simulink library "rfmathmodels1"  (Simulink 6.0)
settings: Solver=ode45  SolverMode=SingleTasking  StartTime=0.0  StopTime=10.0  RelTol=1e-3
undefined symbols (not defined in the file or in its folder): c1, inputGain, kT, method, outputGain
libraries: rfprivate1 x6, dspsigattribs x4, dspmathops x2, dsparch3 x1
settings Model: RequirementInfo=9  CovMetricSettings=d  Creator=tdelve  LastModifiedBy=rzeng  ExtModeAutoUpdateStatusClock=off  ProdHWDeviceType=Specified
settings DataIOCC: SignalLoggingName=logsOut
settings OptimizationCC: BooleanDataType=off
settings DebuggingCC: CheckExecutionContextPreStartOutputMsg=on  CheckExecutionContextRuntimeOutputMsg=on  SolverPrmCheckMsg=none
settings HardwareCC: ProdHWDeviceType=Specified
settings ModelReferenceCC: UpdateModelReferenceTargets=IfOutOfDate
settings SFSimCC: SFSimApplyToAllLibs=on  SFSimBuildMode=Incremental

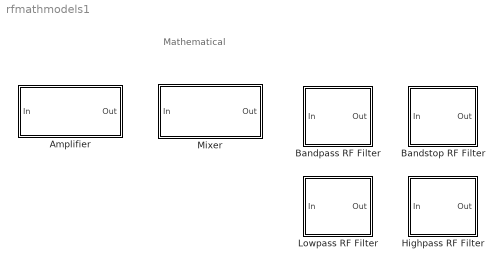
== system rfmathmodels1 ==
  note: Mathematical
  Amplifier : Subsystem  PropExecContextAcrossSSBoundary=on  mask(Amplifier){model_select=Linear, linGaindB=0, GindB=0, iip3=30, am2pm=0, amam=[2.1587 1.1517], ampm=[4.0033 9.1040], x=[8.1081 1.5413 6.5202 -0.0718], y=[4.6645 2.0965 10.88 -0.003], p=0.5, GoutdB=0, vsat=1, method_select=Noise factor, ntemp=290, nfigure=3.01, nfactor=2, seed=67987}
      mask prompts: model_select "Method:"; linGaindB "Linear gain (dB):"; GindB "Input scaling (dB):"; iip3 "IIP3 (dBm):"; am2pm "AM/PM conversion (degrees per dB):"; amam "AM/AM parameters [alpha beta]:"; ampm "AM/PM parameters [alpha beta]:"; x "AM/AM parameters [x1 x2 x3 x4]:"; y "AM/PM parameters [y1 y2 y3 y4]:"; p "Smoothness factor:"; GoutdB "Output scaling (dB):"; vsat "Output saturation level:"; method_select "Specification method:"; ntemp "Noise temperature (K):"; nfigure "Noise figure (dB):"; nfactor "Noise factor:"; seed "Initial seed:"
      mask help:
      | Complex baseband model of amplifier with noise.
      |
      | In addition to Linear amplifier, this block has five different methods to model the nonlinear amplifier.
      |
      | Two of the nonlinear methods (Cubic Polynomial and Hyperbolic Tangent) fit curves to measured data provided by the gain and third order intercept point (IIP3) parameters.
      |
      | The other three nonlinear methods use models originated by Saleh, Ghorbani, and Rapp.  The Saleh and Ghorbani models are based on normalized nonlinear transfer functions.  Use the Input scaling and Output scaling parameters to adjust signal levels up or down from their normalized values.
      |
      | The amount of noise added to the output signal may be specified either in terms of noise temperature, noise figure, or noise factor.
      mask init:
      | [c1, method, inputGain, outputGain, kT] = rfblksmathamp1(gcb, 'rfInit');
      mask Help: helpview(rfbhelp)
      mask StyleString: popup(Linear|Cubic polynomial|Hyperbolic tangent|Saleh model|Ghorbani model|Rapp model),edit,edit,edit,edit,edit,edit,edit,edit,edit,edit,edit,popup(Noise temperature|Noise figure|Noise factor),edit,edit,edit,edit
      mask CallbackString: rfblksmathamp1(gcb, 'rfModel');||||||||||||rfblksmathamp1(gcb, 'rfMethod');||||
      mask Display: disp('Amplifier');
  Bandpass RF Filter : Subsystem  PropExecContextAcrossSSBoundary=on  mask(Bandpass RF Filter){method=Butterworth, filttype=Bandpass, N=3, flo=1.9998e9, fhi=2.0002e9, Rp=1, Rs=10, MaxLength=32, Fc=2e9, Ts=1e-6}
      mask prompts: method "Design method:"; filttype "Filter type:"; N "Filter order:"; flo "Lower passband edge frequency (Hz):"; fhi "Upper passband edge frequency (Hz):"; Rp "Passband ripple in dB:"; Rs "Stopband attenuation in dB:"; MaxLength "Max length of impulse response:"; Fc "Center frequency (Hz):"; Ts "Sample time (s):"
      mask help: Design one of several standard bandpass filters, implemented in baseband equivalent complex form.
      mask init:
      | load rfblksfiltericons;
      | h = [yline+2 yline ywav];
      | w = [xline xline xwav];
      | model = rfblksfilters1(gcb, 'rfInit');
      mask Help: helpview(rfbhelp)
      mask StyleString: popup(Butterworth|Chebyshev I|Chebyshev II|Elliptic|Bessel),popup(Bandpass),edit,edit,edit,edit,edit,edit,edit,edit
      mask CallbackString: rfblksfilters1(gcb);|rfblksfilters1(gcb);||||||||
      mask Display: plot(w,h)
  Bandstop RF Filter : Subsystem  PropExecContextAcrossSSBoundary=on  mask(Bandstop RF Filter){method=Butterworth, filttype=Bandstop, N=3, flo=1.9998e9, fhi=2.0002e9, Rp=1, Rs=10, MaxLength=32, Fc=2e9, Ts=1e-6}
      mask prompts: method "Design method:"; filttype "Filter type:"; N "Filter order:"; flo "Lower passband edge frequency (Hz):"; fhi "Upper passband edge frequency (Hz):"; Rp "Passband ripple in dB:"; Rs "Stopband attenuation in dB:"; MaxLength "Max length of impulse response:"; Fc "Center frequency (Hz):"; Ts "Sample time (s):"
      mask help: Design one of several standard bandstop filters, implemented in baseband equivalent complex form.
      mask init:
      | load rfblksfiltericons;
      | h = [yline+1 ywav];
      | w = [xline xwav];
      | model = rfblksfilters1(gcb, 'rfInit');
      mask Help: helpview(rfbhelp)
      mask StyleString: popup(Butterworth|Chebyshev I|Chebyshev II|Elliptic|Bessel),popup(Bandstop),edit,edit,edit,edit,edit,edit,edit,edit
      mask CallbackString: rfblksfilters1(gcb);|rfblksfilters1(gcb);||||||||
      mask Display: plot(w,h)
  Highpass RF Filter : Subsystem  PropExecContextAcrossSSBoundary=on  mask(Highpass RF Filter){method=Butterworth, filttype=Highpass, N=3, flo=1.9998e9, fhi=2.0002e9, Rp=1, Rs=10, MaxLength=32, Fc=2e9, Ts=1e-6}
      mask prompts: method "Design method:"; filttype "Filter type:"; N "Filter order:"; flo "Passband edge frequency (Hz):"; fhi "(unused)"; Rp "Passband ripple in dB:"; Rs "Stopband attenuation in dB:"; MaxLength "Max length of impulse response:"; Fc "Center frequency:"; Ts "Sample time (s):"
      mask help: Design one of several standard highpass filters, implemented in baseband equivalent complex form.
      mask init:
      | load rfblksfiltericons;
      | h = [yline yline+1 ywav];
      | w = [xline xline xwav];
      | model = rfblksfilters1(gcb, 'rfInit');
      mask Help: helpview(rfbhelp)
      mask StyleString: popup(Butterworth|Chebyshev I|Chebyshev II|Elliptic|Bessel),popup(Highpass),edit,edit,edit,edit,edit,edit,edit,edit
      mask CallbackString: rfblksfilters1(gcb);|rfblksfilters1(gcb);||||||||
      mask Display: plot(w,h)
  Lowpass RF Filter : Subsystem  PropExecContextAcrossSSBoundary=on  mask(Lowpass RF Filter){method=Butterworth, filttype=Lowpass, N=3, flo=1.9998e9, fhi=2.0002e9, Rp=1, Rs=10, MaxLength=32, Fc=2e9, Ts=1e-6}
      mask prompts: method "Design method:"; filttype "Filter type:"; N "Filter order:"; flo "Passband edge frequency (Hz):"; fhi "(unused)"; Rp "Passband ripple in dB:"; Rs "Stopband attenuation in dB:"; MaxLength "Max length of impulse response:"; Fc "Center frequency (Hz):"; Ts "Sample time (s):"
      mask help: Design one of several standard lowpass filters, implemented in baseband equivalent complex form.
      mask init:
      | load rfblksfiltericons;
      | h = [yline+2 yline+1 ywav];
      | w = [xline xline xwav];
      | model = rfblksfilters1(gcb, 'rfInit');
      mask Help: helpview(rfbhelp)
      mask StyleString: popup(Butterworth|Chebyshev I|Chebyshev II|Elliptic|Bessel),popup(Lowpass),edit,edit,edit,edit,edit,edit,edit,edit
      mask CallbackString: rfblksfilters1(gcb);|rfblksfilters1(gcb);||||||||
      mask Display: plot(w,h)
  Mixer : Subsystem  PropExecContextAcrossSSBoundary=on  mask(Mixer){loss=0, PhNs=-120, Fo=100, seed=2137}
      mask prompts: loss "Conversion loss (dB):"; PhNs "Phase noise level (dBc/Hz):"; Fo "Frequency offset (Hz):"; seed "Initial seed:"
      mask help:
      | Complex baseband model of mixer with phase noise.
      |
      | The phase noise of this block characterized by a 1/f slope.  The level of the spectrum is specified by the noise power contained in a one hertz bandwidth offset from the carrier by a certain frequency.
      mask init:
      | c1 = 10^(-loss/20);
      | 
      | if PhNs>0,
      | 	error('Phase noise level should be negative.');
      | end
      | num = sqrt(2*pi*Fo*10^((PhNs)/10));
      | if num>.1,
      | 	warning('Current parameters in phase noise block may produce inaccurate results.');
      | end
      | num_taps = 64;
      | den = zeros(1,num_taps);
      | den(1) = 1;
      | for idx = 2:num_taps
      |    den(idx) = (idx - 2.5) * den(idx-1) / (idx-1);
      | end
      mask Help: helpview(rfbhelp)
      mask Display: disp('Mixer');

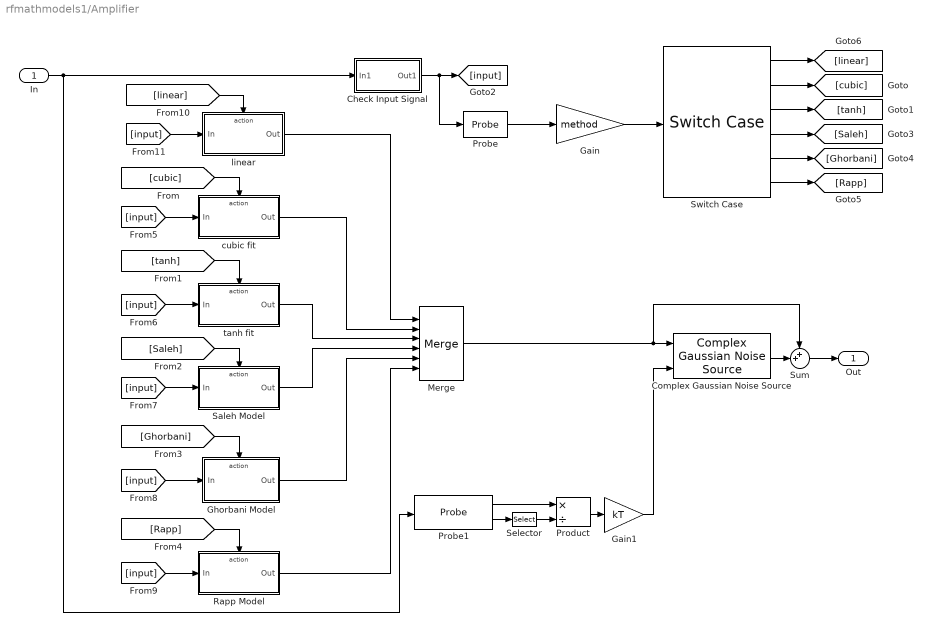
== system rfmathmodels1/Amplifier ==
  In : Inport  LatchInput=off
  Check Input Signal : Subsystem  PropExecContextAcrossSSBoundary=on
      mask Display: disp('Check\nInput Signal');
  Complex Gaussian Noise Source : rfprivate1/Complex Gaussian Noise Source
  Gain : Gain  Gain=method  SaturateOnIntegerOverflow=on
  Gain1 : Gain  Gain=kT  SaturateOnIntegerOverflow=on
  Ghorbani Model : Subsystem  TreatAsAtomicUnit=on  PropExecContextAcrossSSBoundary=on
  Merge : Merge  Inputs=6
  Probe : Probe  ProbeWidth=off  ProbeSampleTime=off
  Probe1 : Probe  ProbeComplexSignal=off
  Product : Product  Inputs=*/  SaturateOnIntegerOverflow=on  InputSameDT=on
  Rapp Model : Subsystem  TreatAsAtomicUnit=on  PropExecContextAcrossSSBoundary=on
  Saleh Model : Subsystem  TreatAsAtomicUnit=on  PropExecContextAcrossSSBoundary=on
  Selector : Selector  InputPortWidth=2
  Sum : Sum  Inputs=++|
  Switch Case : SwitchCase  CaseConditions={0 1 2 3 4 5}  CaseShowDefault=off
  cubic fit : Subsystem  TreatAsAtomicUnit=on  PropExecContextAcrossSSBoundary=on
  linear : Subsystem  TreatAsAtomicUnit=on  PropExecContextAcrossSSBoundary=on
  tanh fit : Subsystem  TreatAsAtomicUnit=on  PropExecContextAcrossSSBoundary=on
  Out : Outport
  wires:
  Merge/1 -> Complex Gaussian Noise Source/1, Sum/1
  Selector/1 -> Product/2
  Probe1/2 -> Selector/1
  Gain1/1 -> Complex Gaussian Noise Source/2
  Product/1 -> Gain1/1
  Probe1/1 -> Product/1
  Sum/1 -> Out/1
  Gain/1 -> Switch Case/1
  [cubic] -> cubic fit/Action
  [tanh] -> tanh fit/Action
  In/1 -> Probe1/1, Check Input Signal/1(In1)
  Check Input Signal/1(Out1) -> [input], Probe/1
  [Rapp] -> Rapp Model/Action
  [Ghorbani] -> Ghorbani Model/Action
  [Saleh] -> Saleh Model/Action
  [input] -> cubic fit/1(In)
  [input] -> Rapp Model/1(In)
  [input] -> Ghorbani Model/1(In)
  [input] -> Saleh Model/1(In)
  [input] -> tanh fit/1(In)
  Probe/1 -> Gain/1
  Rapp Model/1(Out) -> Merge/6
  [linear] -> linear/Action
  [input] -> linear/1(In)
  Ghorbani Model/1(Out) -> Merge/5
  Saleh Model/1(Out) -> Merge/4
  tanh fit/1(Out) -> Merge/3
  cubic fit/1(Out) -> Merge/2
  linear/1(Out) -> Merge/1
  Switch Case/6 -> [Rapp]
  Switch Case/2 -> [cubic]
  Switch Case/3 -> [tanh]
  Switch Case/4 -> [Saleh]
  Switch Case/5 -> [Ghorbani]
  Switch Case/1 -> [linear]
  Complex Gaussian Noise Source/1 -> Sum/2

== system rfmathmodels1/Bandpass RF Filter ==
  In : Inport  LatchInput=off
  RF Filter : rfprivate1/RF Filter  model=model  Ts=Ts
  Out : Outport
  wires:
  In/1 -> RF Filter/1
  RF Filter/1 -> Out/1

== system rfmathmodels1/Bandstop RF Filter ==
  In : Inport  LatchInput=off
  RF Filter : rfprivate1/RF Filter  model=model  Ts=Ts
  Out : Outport
  wires:
  In/1 -> RF Filter/1
  RF Filter/1 -> Out/1

== system rfmathmodels1/Highpass RF Filter ==
  In : Inport  LatchInput=off
  RF Filter : rfprivate1/RF Filter  model=model  Ts=Ts
  Out : Outport
  wires:
  In/1 -> RF Filter/1
  RF Filter/1 -> Out/1

== system rfmathmodels1/Lowpass RF Filter ==
  In : Inport  LatchInput=off
  RF Filter : rfprivate1/RF Filter  model=model  Ts=Ts
  Out : Outport
  wires:
  In/1 -> RF Filter/1
  RF Filter/1 -> Out/1

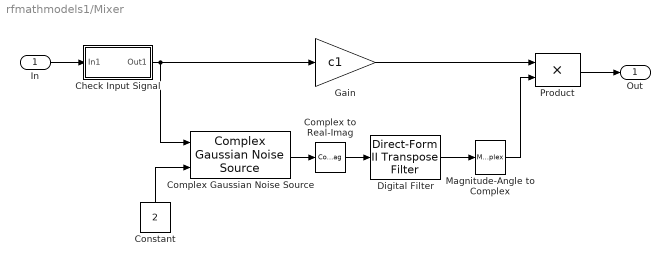
== system rfmathmodels1/Mixer ==
  In : Inport  LatchInput=off
  Check Input Signal : Subsystem  PropExecContextAcrossSSBoundary=on
      mask Display: disp('Check\nInput Signal');
  Complex Gaussian Noise Source : rfprivate1/Complex Gaussian Noise Source
  Complex to Real-Imag : ComplexToRealImag  Output=Real
  Constant : Constant  Orientation=up  Value=2  SampleTime=Inf
  Digital Filter : dsparch3/Direct-Form II Transpose Filter  num=num  den=den  ic=0
  Gain : Gain  Gain=c1  SaturateOnIntegerOverflow=on
  Magnitude-Angle to Complex : MagnitudeAngleToComplex  Input=Angle  ConstantPart=1
  Product : Product  SaturateOnIntegerOverflow=on  InputSameDT=on
  Out : Outport
  wires:
  Digital Filter/1 -> Magnitude-Angle to Complex/1
  Magnitude-Angle to Complex/1 -> Product/2
  Complex to Real-Imag/1 -> Digital Filter/1
  Product/1 -> Out/1
  In/1 -> Check Input Signal/1(In1)
  Check Input Signal/1(Out1) -> Gain/1, Complex Gaussian Noise Source/1
  Gain/1 -> Product/1
  Complex Gaussian Noise Source/1 -> Complex to Real-Imag/1
  Constant/1 -> Complex Gaussian Noise Source/2

== system rfmathmodels1/Amplifier/Check Input Signal ==
  In1 : Inport  LatchInput=off
  Check Signal Attributes : dspsigattribs/Check Signal Attributes  SigAttribCheckMethod=Does not match attributes exactly  Complexity=Complex  Frame=Ignore  DimsCheckMethod=Is...  Dimensions=Column vector (2-D) or scalar  DatatypeCheckMethod=Ignore  DatatypeGeneral=Boolean  DtypeFloatSpecific=Any floating-point  DtypeFixedSpecific=Any fixed-point  DtypeIntSpecific=Any integer  SampleMode=Ignore
  Check Signal Attributes1 : dspsigattribs/Check Signal Attributes  SigAttribCheckMethod=Matches attributes exactly  Complexity=Ignore  Frame=Sample-based  DimsCheckMethod=Is...  Dimensions=Vector (1-D or 2-D)  DatatypeCheckMethod=Ignore  DatatypeGeneral=Boolean  DtypeFloatSpecific=Any floating-point  DtypeFixedSpecific=Any fixed-point  DtypeIntSpecific=Any integer  SampleMode=Ignore
  Out1 : Outport
  wires:
  In1/1 -> Check Signal Attributes/1
  Check Signal Attributes1/1 -> Out1/1
  Check Signal Attributes/1 -> Check Signal Attributes1/1

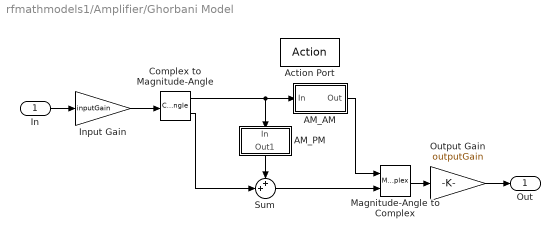
== system rfmathmodels1/Amplifier/Ghorbani Model ==
  In : Inport  LatchInput=off
  Action Port : ActionPort
  AM_AM : Subsystem  PropExecContextAcrossSSBoundary=on
      mask Display: disp('AM/AM')
  AM_PM : Subsystem  Orientation=down  PropExecContextAcrossSSBoundary=on
      mask Display: disp('AM/PM')
  Complex to Magnitude-Angle : ComplexToMagnitudeAngle
  Input Gain : Gain  Gain=inputGain  SaturateOnIntegerOverflow=on
  Magnitude-Angle to Complex : MagnitudeAngleToComplex
  Output Gain : Gain  Gain=outputGain  SaturateOnIntegerOverflow=on
  Sum : Sum  Inputs=++|  SaturateOnIntegerOverflow=on  InputSameDT=on
  Out : Outport
  wires:
  Sum/1 -> Magnitude-Angle to Complex/2
  AM_PM/1(Out1) -> Sum/1
  Output Gain/1 -> Out/1
  In/1 -> Input Gain/1
  Complex to Magnitude-Angle/2 -> Sum/2
  Input Gain/1 -> Complex to Magnitude-Angle/1
  Magnitude-Angle to Complex/1 -> Output Gain/1
  AM_AM/1(Out) -> Magnitude-Angle to Complex/1
  Complex to Magnitude-Angle/1 -> AM_AM/1(In), AM_PM/1(In)

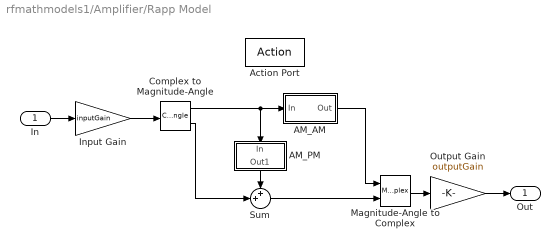
== system rfmathmodels1/Amplifier/Rapp Model ==
  In : Inport  LatchInput=off
  Action Port : ActionPort
  AM_AM : Subsystem  PropExecContextAcrossSSBoundary=on
      mask Display: disp('AM/AM')
  AM_PM : Subsystem  Orientation=down  PropExecContextAcrossSSBoundary=on
      mask Display: disp('AM/PM')
  Complex to Magnitude-Angle : ComplexToMagnitudeAngle
  Input Gain : Gain  Gain=inputGain  SaturateOnIntegerOverflow=on
  Magnitude-Angle to Complex : MagnitudeAngleToComplex
  Output Gain : Gain  Gain=outputGain  SaturateOnIntegerOverflow=on
  Sum : Sum  Inputs=++|  SaturateOnIntegerOverflow=on  InputSameDT=on
  Out : Outport
  wires:
  Output Gain/1 -> Out/1
  In/1 -> Input Gain/1
  Input Gain/1 -> Complex to Magnitude-Angle/1
  Magnitude-Angle to Complex/1 -> Output Gain/1
  AM_AM/1(Out) -> Magnitude-Angle to Complex/1
  Complex to Magnitude-Angle/1 -> AM_AM/1(In), AM_PM/1(In)
  AM_PM/1(Out1) -> Sum/1
  Complex to Magnitude-Angle/2 -> Sum/2
  Sum/1 -> Magnitude-Angle to Complex/2

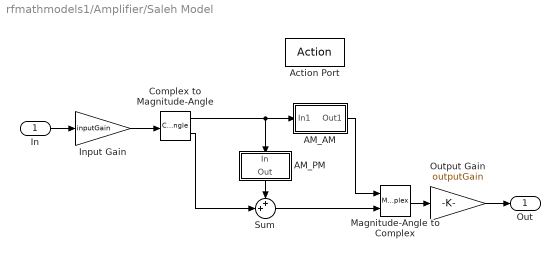
== system rfmathmodels1/Amplifier/Saleh Model ==
  In : Inport  LatchInput=off
  Action Port : ActionPort
  AM_AM : Subsystem  PropExecContextAcrossSSBoundary=on
      mask Display: disp('AM/AM')
  AM_PM : Subsystem  Orientation=down  PropExecContextAcrossSSBoundary=on
      mask Display: disp('AM/PM')
  Complex to Magnitude-Angle : ComplexToMagnitudeAngle
  Input Gain : Gain  Gain=inputGain  SaturateOnIntegerOverflow=on
  Magnitude-Angle to Complex : MagnitudeAngleToComplex
  Output Gain : Gain  Gain=outputGain  SaturateOnIntegerOverflow=on
  Sum : Sum  Inputs=++|  SaturateOnIntegerOverflow=on  InputSameDT=on
  Out : Outport
  wires:
  Sum/1 -> Magnitude-Angle to Complex/2
  AM_PM/1(Out) -> Sum/1
  Output Gain/1 -> Out/1
  In/1 -> Input Gain/1
  Complex to Magnitude-Angle/2 -> Sum/2
  Input Gain/1 -> Complex to Magnitude-Angle/1
  Magnitude-Angle to Complex/1 -> Output Gain/1
  AM_AM/1(Out1) -> Magnitude-Angle to Complex/1
  Complex to Magnitude-Angle/1 -> AM_AM/1(In1), AM_PM/1(In)

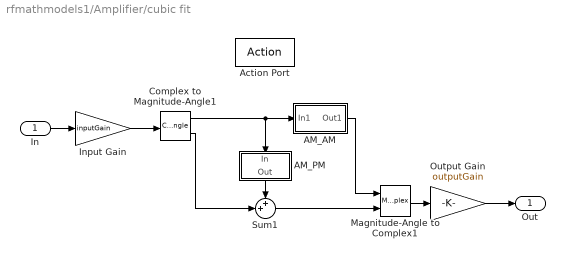
== system rfmathmodels1/Amplifier/cubic fit ==
  In : Inport  LatchInput=off
  Action Port : ActionPort
  AM_AM : Subsystem  PropExecContextAcrossSSBoundary=on
      mask Display: disp('AM/AM')
  AM_PM : Subsystem  Orientation=down  PropExecContextAcrossSSBoundary=on
      mask Display: disp('AM/PM')
  Complex to Magnitude-Angle1 : ComplexToMagnitudeAngle
  Input Gain : Gain  Gain=inputGain  SaturateOnIntegerOverflow=on
  Magnitude-Angle to Complex1 : MagnitudeAngleToComplex
  Output Gain : Gain  Gain=outputGain  SaturateOnIntegerOverflow=on
  Sum1 : Sum  Inputs=++|  SaturateOnIntegerOverflow=on  InputSameDT=on
  Out : Outport
  wires:
  Complex to Magnitude-Angle1/1 -> AM_AM/1(In1), AM_PM/1(In)
  AM_AM/1(Out1) -> Magnitude-Angle to Complex1/1
  Magnitude-Angle to Complex1/1 -> Output Gain/1
  Input Gain/1 -> Complex to Magnitude-Angle1/1
  Complex to Magnitude-Angle1/2 -> Sum1/2
  In/1 -> Input Gain/1
  Output Gain/1 -> Out/1
  AM_PM/1(Out) -> Sum1/1
  Sum1/1 -> Magnitude-Angle to Complex1/2

== system rfmathmodels1/Amplifier/linear ==
  In : Inport  LatchInput=off
  Action Port : ActionPort
  Gain : Gain  Gain=c1  SaturateOnIntegerOverflow=on
  Out : Outport
  wires:
  In/1 -> Gain/1
  Gain/1 -> Out/1

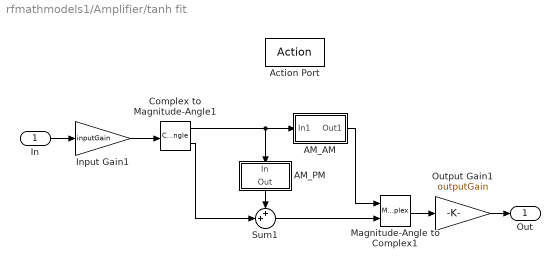
== system rfmathmodels1/Amplifier/tanh fit ==
  In : Inport  LatchInput=off
  Action Port : ActionPort
  AM_AM : Subsystem  PropExecContextAcrossSSBoundary=on
      mask Display: disp('AM/AM')
  AM_PM : Subsystem  Orientation=down  PropExecContextAcrossSSBoundary=on
      mask Display: disp('AM/PM')
  Complex to Magnitude-Angle1 : ComplexToMagnitudeAngle
  Input Gain1 : Gain  Gain=inputGain  SaturateOnIntegerOverflow=on
  Magnitude-Angle to Complex1 : MagnitudeAngleToComplex
  Output Gain1 : Gain  Gain=outputGain  SaturateOnIntegerOverflow=on
  Sum1 : Sum  Inputs=++|  SaturateOnIntegerOverflow=on  InputSameDT=on
  Out : Outport
  wires:
  Complex to Magnitude-Angle1/1 -> AM_AM/1(In1), AM_PM/1(In)
  AM_AM/1(Out1) -> Magnitude-Angle to Complex1/1
  Magnitude-Angle to Complex1/1 -> Output Gain1/1
  Input Gain1/1 -> Complex to Magnitude-Angle1/1
  Complex to Magnitude-Angle1/2 -> Sum1/2
  In/1 -> Input Gain1/1
  Output Gain1/1 -> Out/1
  AM_PM/1(Out) -> Sum1/1
  Sum1/1 -> Magnitude-Angle to Complex1/2

== system rfmathmodels1/Mixer/Check Input Signal ==
  In1 : Inport  LatchInput=off
  Check Signal Attributes : dspsigattribs/Check Signal Attributes  SigAttribCheckMethod=Does not match attributes exactly  Complexity=Complex  Frame=Ignore  DimsCheckMethod=Is...  Dimensions=Column vector (2-D) or scalar  DatatypeCheckMethod=Ignore  DatatypeGeneral=Boolean  DtypeFloatSpecific=Any floating-point  DtypeFixedSpecific=Any fixed-point  DtypeIntSpecific=Any integer  SampleMode=Ignore
  Check Signal Attributes1 : dspsigattribs/Check Signal Attributes  SigAttribCheckMethod=Matches attributes exactly  Complexity=Ignore  Frame=Sample-based  DimsCheckMethod=Is...  Dimensions=Vector (1-D or 2-D)  DatatypeCheckMethod=Ignore  DatatypeGeneral=Boolean  DtypeFloatSpecific=Any floating-point  DtypeFixedSpecific=Any fixed-point  DtypeIntSpecific=Any integer  SampleMode=Ignore
  Out1 : Outport
  wires:
  Check Signal Attributes/1 -> Check Signal Attributes1/1
  Check Signal Attributes1/1 -> Out1/1
  In1/1 -> Check Signal Attributes/1

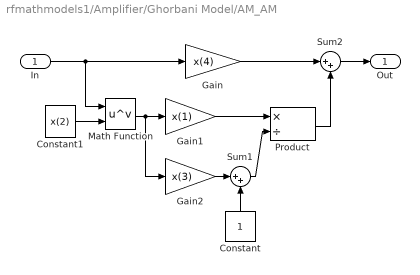
== system rfmathmodels1/Amplifier/Ghorbani Model/AM_AM ==
  In : Inport  LatchInput=off
  Constant : Constant  Orientation=up
  Constant1 : Constant  Value=x(2)
  Gain : Gain  Gain=x(4)  SaturateOnIntegerOverflow=on
  Gain1 : Gain  Gain=x(1)  SaturateOnIntegerOverflow=on
  Gain2 : Gain  Gain=x(3)  SaturateOnIntegerOverflow=on
  Math Function : Math  Operator=pow  SaturateOnIntegerOverflow=on
  Product : Product  Inputs=*/  SaturateOnIntegerOverflow=on  InputSameDT=on
  Sum1 : Sum  Inputs=|++  SaturateOnIntegerOverflow=on  InputSameDT=on
  Sum2 : Sum  Inputs=|++  SaturateOnIntegerOverflow=on  InputSameDT=on
  Out : Outport
  wires:
  Sum2/1 -> Out/1
  In/1 -> Math Function/1, Gain/1
  Sum1/1 -> Product/2
  Gain2/1 -> Sum1/1
  Constant/1 -> Sum1/2
  Product/1 -> Sum2/2
  Gain1/1 -> Product/1
  Constant1/1 -> Math Function/2
  Math Function/1 -> Gain2/1, Gain1/1
  Gain/1 -> Sum2/1

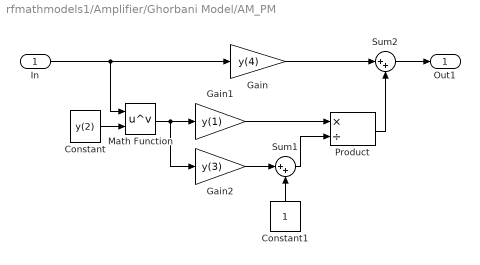
== system rfmathmodels1/Amplifier/Ghorbani Model/AM_PM ==
  In : Inport  LatchInput=off
  Constant : Constant  Value=y(2)
  Constant1 : Constant  Orientation=up
  Gain : Gain  Gain=y(4)  SaturateOnIntegerOverflow=on
  Gain1 : Gain  Gain=y(1)  SaturateOnIntegerOverflow=on
  Gain2 : Gain  Gain=y(3)  SaturateOnIntegerOverflow=on
  Math Function : Math  Operator=pow  SaturateOnIntegerOverflow=on
  Product : Product  Inputs=*/  SaturateOnIntegerOverflow=on  InputSameDT=on
  Sum1 : Sum  Inputs=|++  SaturateOnIntegerOverflow=on  InputSameDT=on
  Sum2 : Sum  Inputs=|++  SaturateOnIntegerOverflow=on  InputSameDT=on
  Out1 : Outport
  wires:
  Sum2/1 -> Out1/1
  In/1 -> Gain/1, Math Function/1
  Sum1/1 -> Product/2
  Gain2/1 -> Sum1/1
  Constant1/1 -> Sum1/2
  Product/1 -> Sum2/2
  Gain1/1 -> Product/1
  Constant/1 -> Math Function/2
  Math Function/1 -> Gain1/1, Gain2/1
  Gain/1 -> Sum2/1

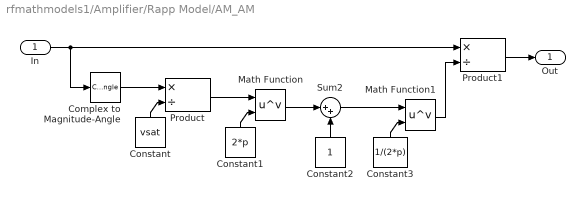
== system rfmathmodels1/Amplifier/Rapp Model/AM_AM ==
  In : Inport  LatchInput=off
  Complex to Magnitude-Angle : ComplexToMagnitudeAngle  Output=Magnitude
  Constant : Constant  Orientation=up  Value=vsat
  Constant1 : Constant  Orientation=up  Value=2*p
  Constant2 : Constant  Orientation=up
  Constant3 : Constant  Orientation=up  Value=1/(2*p)
  Math Function : Math  Operator=pow  SaturateOnIntegerOverflow=on
  Math Function1 : Math  Operator=pow  SaturateOnIntegerOverflow=on
  Product : Product  Inputs=*/  SaturateOnIntegerOverflow=on  InputSameDT=on
  Product1 : Product  Inputs=*/  SaturateOnIntegerOverflow=on  InputSameDT=on
  Sum2 : Sum  Inputs=|++  SaturateOnIntegerOverflow=on  InputSameDT=on
  Out : Outport
  wires:
  Product1/1 -> Out/1
  In/1 -> Product1/1, Complex to Magnitude-Angle/1
  Constant/1 -> Product/2
  Constant2/1 -> Sum2/2
  Product/1 -> Math Function/1
  Math Function/1 -> Sum2/1
  Constant1/1 -> Math Function/2
  Complex to Magnitude-Angle/1 -> Product/1
  Sum2/1 -> Math Function1/1
  Constant3/1 -> Math Function1/2
  Math Function1/1 -> Product1/2

== system rfmathmodels1/Amplifier/Rapp Model/AM_PM ==
  In : Inport  LatchInput=off
  Ground : Ground
  Terminator : Terminator
  Out1 : Outport
  wires:
  In/1 -> Terminator/1
  Ground/1 -> Out1/1

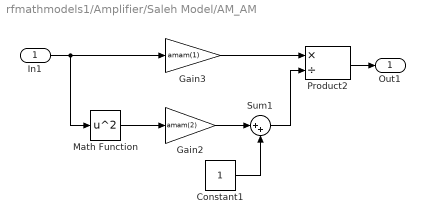
== system rfmathmodels1/Amplifier/Saleh Model/AM_AM ==
  In1 : Inport  LatchInput=off
  Constant1 : Constant
  Gain2 : Gain  Gain=amam(2)  SaturateOnIntegerOverflow=on
  Gain3 : Gain  Gain=amam(1)  SaturateOnIntegerOverflow=on
  Math Function : Math  Operator=square  SaturateOnIntegerOverflow=on
  Product2 : Product  Inputs=*/  SaturateOnIntegerOverflow=on  InputSameDT=on
  Sum1 : Sum  Inputs=|++  SaturateOnIntegerOverflow=on  InputSameDT=on
  Out1 : Outport
  wires:
  Product2/1 -> Out1/1
  In1/1 -> Gain3/1, Math Function/1
  Gain3/1 -> Product2/1
  Sum1/1 -> Product2/2
  Constant1/1 -> Sum1/2
  Gain2/1 -> Sum1/1
  Math Function/1 -> Gain2/1

== system rfmathmodels1/Amplifier/Saleh Model/AM_PM ==
  In : Inport  LatchInput=off
  Constant : Constant  Orientation=up
  Gain : Gain  Gain=ampm(2)  SaturateOnIntegerOverflow=on
  Gain1 : Gain  Gain=ampm(1)  SaturateOnIntegerOverflow=on
  Math Function : Math  Operator=square  SaturateOnIntegerOverflow=on
  Product : Product  Inputs=*/  SaturateOnIntegerOverflow=on  InputSameDT=on
  Sum : Sum  Inputs=|++  SaturateOnIntegerOverflow=on  InputSameDT=on
  Out : Outport
  wires:
  In/1 -> Math Function/1
  Math Function/1 -> Gain/1, Gain1/1
  Product/1 -> Out/1
  Gain/1 -> Sum/1
  Constant/1 -> Sum/2
  Sum/1 -> Product/2
  Gain1/1 -> Product/1

== system rfmathmodels1/Amplifier/cubic fit/AM_AM ==
  In1 : Inport  LatchInput=off
  Constant : Constant  Value=3
  Gain : Gain  Gain=1/3  SaturateOnIntegerOverflow=on
  Math Function : Math  Operator=pow  SaturateOnIntegerOverflow=on
  Saturation I : Saturate  UpperLimit=1  LowerLimit=-1
  Sum : Sum  Inputs=+-|  SaturateOnIntegerOverflow=on  InputSameDT=on
  Out1 : Outport
  wires:
  Sum/1 -> Out1/1
  Saturation I/1 -> Math Function/1, Sum/1
  Math Function/1 -> Gain/1
  Constant/1 -> Math Function/2
  Gain/1 -> Sum/2
  In1/1 -> Saturation I/1

== system rfmathmodels1/Amplifier/cubic fit/AM_PM ==
  In : Inport  LatchInput=off
  Input Gain : Gain  Gain=am2pm*pi/180  SaturateOnIntegerOverflow=on
  dB Conversion : dspmathops/dB Conversion  dBtype=dB  intype=Amplitude  R=1  fuzz=on
  Out : Outport
  wires:
  In/1 -> dB Conversion/1
  Input Gain/1 -> Out/1
  dB Conversion/1 -> Input Gain/1

== system rfmathmodels1/Amplifier/tanh fit/AM_AM ==
  In1 : Inport  LatchInput=off
  Trigonometric Function : Trigonometry  Operator=tanh
  Out1 : Outport
  wires:
  Trigonometric Function/1 -> Out1/1
  In1/1 -> Trigonometric Function/1

== system rfmathmodels1/Amplifier/tanh fit/AM_PM ==
  In : Inport  LatchInput=off
  Input Gain : Gain  Gain=am2pm*pi/180  SaturateOnIntegerOverflow=on
  dB Conversion : dspmathops/dB Conversion  dBtype=dB  intype=Amplitude  R=1  fuzz=on
  Out : Outport
  wires:
  In/1 -> dB Conversion/1
  dB Conversion/1 -> Input Gain/1
  Input Gain/1 -> Out/1
